simulink model "master_task"  (Simulink 3.00)
libraries: mathlib x12

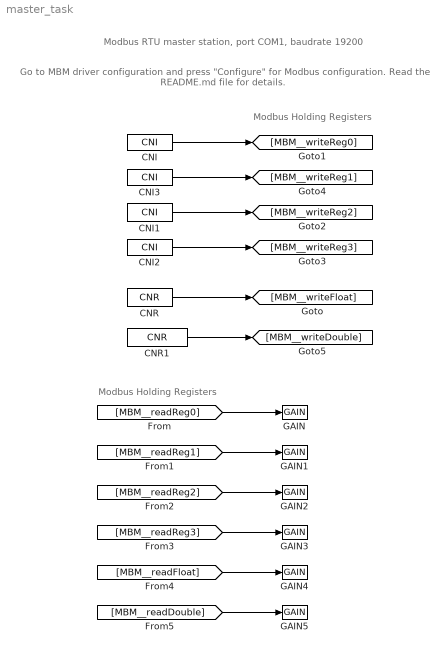
== system master_task ==
  note: Modbus RTU master station, port COM1, baudrate 19200
  note: Modbus Holding Registers
  note: Modbus Holding Registers
  note: Go to MBM driver configuration and press "Configure" for Modbus configuration.
      |
      | Read the README.md file for details.
  CNI : mathlib/CNI  icn=111
  CNI1 : mathlib/CNI  icn=64917
  CNI2 : mathlib/CNI  icn=-29999
  CNI3 : mathlib/CNI  icn=-95
  CNR : mathlib/CNR  ycn=-78.57
  CNR1 : mathlib/CNR  ycn=-79315.18
  GAIN{,1..5} (6 alike) : mathlib/GAIN  k=1
  wires:
  CNI/1 -> [MBM__writeReg0]
  CNI1/1 -> [MBM__writeReg2]
  CNI2/1 -> [MBM__writeReg3]
  CNI3/1 -> [MBM__writeReg1]
  CNR/1 -> [MBM__writeFloat]
  CNR1/1 -> [MBM__writeDouble]
  [MBM__readReg0] -> GAIN/1
  [MBM__readReg1] -> GAIN1/1
  [MBM__readReg2] -> GAIN2/1
  [MBM__readReg3] -> GAIN3/1
  [MBM__readFloat] -> GAIN4/1
  [MBM__readDouble] -> GAIN5/1
